simulink model "template_inverted_pendulum_2021b"  (R2021b)
settings: Solver=FixedStepDiscrete  StartTime=0.0  StopTime=inf  FixedStep=0.005  RelTol=1e-3
values from neighbouring files (symbols this model uses):
  LPF_A = [0              1           0               0 ... (first row only)    [IP_experiment.m]    (also in IP_sim.m)
  LPF_B = [                    0                           0 ... (first row only)    [IP_experiment.m]    (also in IP_sim.m)
  LPF_C = [-1/T_s    1/T_s         0         0 ... (first row only)    [IP_experiment.m]    (also in IP_sim.m)
  LPF_D = zeros(2)    [IP_experiment.m]    (also in IP_sim.m)
  rnd = randi(500, 1)    [IP_experiment.m]    (also in IP_sim.m)
  xd = [0.3          0.0      0   0]'    [IP.m]    (also in IP_experiment.m = [0.0    0.0]; IP_sim.m = sp(1:12800, 1))
undefined symbols (not defined in the file or in its folder): K, National_Instruments, PCI
libraries: sldrtlib x2, simulink_extras x1
settings Model: SimulationMode=external  ExtModeTrigDuration=200000  Creator=magudelo  LastModifiedBy=yz
settings SolverCC: AlgebraicLoopSolver=TrustRegion  InsertRTBMode=Always
settings DataIOCC: LimitDataPoints=on  SaveFormat=Array  SignalLoggingSaveFormat=ModelDataLogs  ReturnWorkspaceOutputs=off
settings OptimizationCC: ExpressionDepthLimit=2147483647
settings DebuggingCC: UnderspecifiedInitializationDetection=Classic  MergeDetectMultiDrivingBlocksExec=none  SolverPrmCheckMsg=warning  FcnCallInpInsideContextMsg=warning  StateNameClashWarn=warning  SFUnexpectedBacktrackingDiag=warning  SFNoUnconditionalDefaultTransitionDiag=warning  SFExecutionAtInitializationDiag=none  SFMachineParentedDataDiag=warning  ArithmeticOperatorsInVariantConditions=warning
settings ModelReferenceCC: PropagateSignalLabelsOutOfModel=off
settings SFSimCC: SimUseLocalCustomCode=off  CustomCodeUndefinedFunction=UseInterfaceOnly
settings RTWCC: Description=Simulink Desktop Real-Time  SystemTargetFile=sldrt.tlc  TemplateMakefile=sldrt.tmf  RTWUseLocalCustomCode=off  RTWCompilerOptimization=on
settings CodeAppCC: MaxIdLength=95  StateflowObjectComments=on
settings SimulinkDesktopRealTimeCC: TargetPreCompLibLocation=C:\Program Files\MATLAB\R2021b\toolbox\sldrt\lib\win64  TargetLangStandard=C89/C90 (ANSI)  SupportVariableSizeSignals=off
settings ConfigComp: CovMetricSettings=dw  CovSaveCumulativeToWorkspaceVar=on  CovSaveSingleToWorkspaceVar=on  CovExternalEMLEnable=off

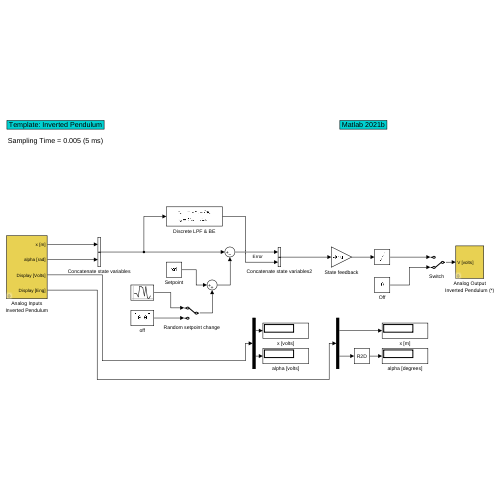
[thumbnail: Simulink's stored preview of the top-level diagram]
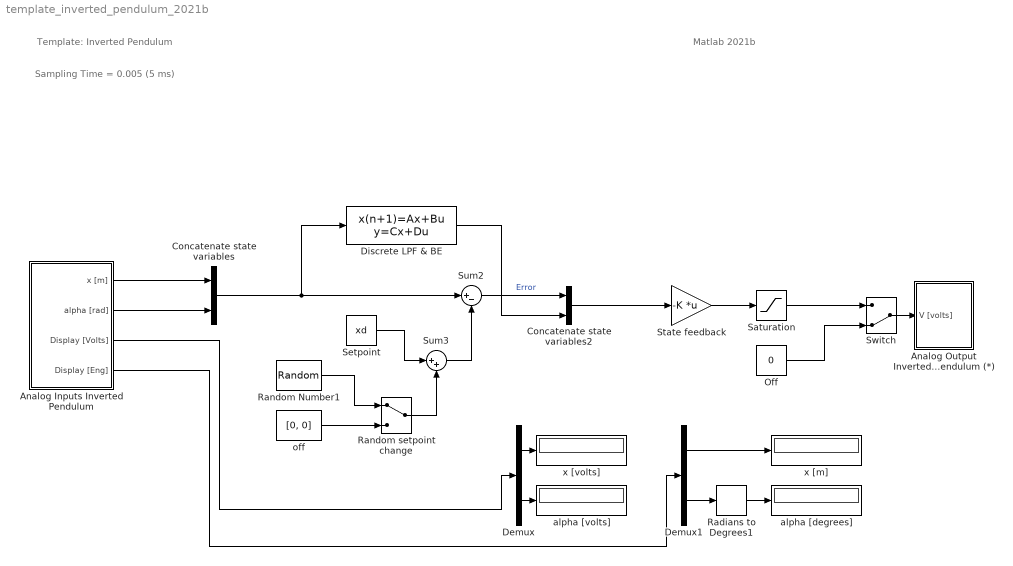
== system template_inverted_pendulum_2021b ==
  note: Matlab 2021b
  note: Template: Inverted Pendulum
  note: Sampling Time = 0.005 (5 ms)
  Analog Inputs Inverted Pendulum : Subsystem  mask(Analog Inputs. Inverted Pendulum){v2m=0.1033, offset_x=0, v2r=0.2482, offset_alfa=0.17011}
      mask prompts: v2m "F_x = Convertion factor from Volts to Meters:"; offset_x "Off_x = Offset for the Cart Position [Volts] :"; v2r "F_alpha = Convertion Factor from Volts to Radians :"; offset_alfa "Off_alpha = Offset for the angle of the rob [Volts] :"
      mask help:
      | Remember:
      |    Cart Position (x)           => channel ACH0
      |    Angle of the rod (alpha) => channel ACH1
      |
      |   Cart Position [m] = F_x * ( Cart Position [v] + off_x )
      |   Angle of the rod [rad] = F_alpha * ( Angle of the rod [v] + off_alpha )
  Analog Output Inverted Pendulum (*) : Subsystem  mask(Analog Output - Inverted Pendulum){}
      mask help:
      | Remember
      |    AO 0 => Power Amplifier + Motor
  Concatenate state variables : Concatenate
  Concatenate state variables2 : Concatenate
  Demux : Demux  Outputs=2
  Demux1 : Demux  Outputs=2
  Discrete LPF & BE : DiscreteStateSpace  A=LPF_A  B=LPF_B  C=LPF_C  D=LPF_D  InitialCondition=[0,0,0,0]  SampleTime=-1
  Off : Constant  Value=0
  Radians to Degrees1 : simulink_extras/Transformations/Radians to Degrees
  Random Number1 : RandomNumber  Mean=[0, 0]  Variance=[0.01, 0]  Seed=rnd  SampleTime=8
  Random setpoint change : ManualSwitch
  Saturation : Saturate  UpperLimit=5  LowerLimit=-5
  Setpoint : Constant  Value=xd
  State feedback : Gain  Gain=-K  Multiplication=Matrix(K*u)
  Sum2 : Sum  Inputs=|+-
  Sum3 : Sum  Inputs=|++
  "Switch  " : ManualSwitch  CurrentSetting=0
  alpha [degrees] : Display
  alpha [volts] : Display
  off : Constant  Value=[0, 0]
  x [m] : Display
  x [volts] : Display
  wires:
  Off/1 -> "Switch  "/2
  Demux/1 -> x [volts]/1
  Demux1/1 -> x [m]/1
  Demux1/2 -> Radians to Degrees1/1
  Radians to Degrees1/1 -> alpha [degrees]/1
  Analog Inputs Inverted Pendulum/4(Display [Eng]) -> Demux1/1
  Demux/2 -> alpha [volts]/1
  Analog Inputs Inverted Pendulum/3(Display [Volts]) -> Demux/1
  Analog Inputs Inverted Pendulum/1(x [m]) -> Concatenate state variables/1
  Concatenate state variables/1 -> Discrete LPF & BE/1, Sum2/1
  Random setpoint change/1 -> Sum3/2
  off/1 -> Random setpoint change/2
  Setpoint/1 -> Sum3/1
  Random Number1/1 -> Random setpoint change/1
  Sum2/1 -> Concatenate state variables2/1  "Error"
  Sum3/1 -> Sum2/2
  Discrete LPF & BE/1 -> Concatenate state variables2/2
  Concatenate state variables2/1 -> State feedback/1
  "Switch  "/1 -> Analog Output Inverted Pendulum (*)/1(V [volts])
  Analog Inputs Inverted Pendulum/2(alpha [rad]) -> Concatenate state variables/2
  Saturation/1 -> "Switch  "/1
  State feedback/1 -> Saturation/1

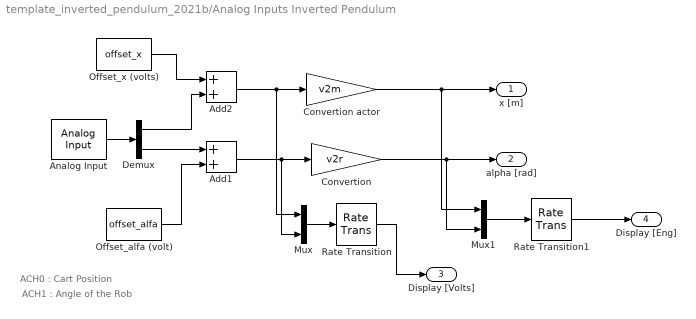
== system template_inverted_pendulum_2021b/Analog Inputs Inverted Pendulum ==
  note: ACH0 : Cart Position
  note: ACH1 : Angle of the Rob
  Add1 : Sum
  Add2 : Sum
  Analog Input : sldrtlib/Analog Input  SampleTime=0.005  MaxMissedTicks=10  ShowMissedTicks=off  YieldWhenWaiting=off  DrvName=National_Instruments/PCI-6014  DrvAddress=4294967295  DrvOptions=[1 0 0 0 0 0]  Channels=[1 2]  RangeMode=1  VoltRange=1  DataType=1
      settings: AttributesFormatString=National Instruments\nPCI-6014 [auto]
  "Convertion " : Gain  Gain=v2r
  Convertion actor : Gain  Gain=v2m
  Demux : Demux  Outputs=2
  Mux : Mux  Inputs=2
  Mux1 : Mux  Inputs=2
  Offset_alfa (volt) : Constant  Value=offset_alfa
  Offset_x (volts) : Constant  Value=offset_x
  Rate Transition : RateTransition  OutPortSampleTime=0.25
  Rate Transition1 : RateTransition  OutPortSampleTime=0.25
  x [m] : Outport  VectorParamsAs1DForOutWhenUnconnected=off
  alpha [rad] : Outport  Port=2  VectorParamsAs1DForOutWhenUnconnected=off
  Display [Volts] : Outport  Port=3  VectorParamsAs1DForOutWhenUnconnected=off
  Display [Eng] : Outport  Port=4  VectorParamsAs1DForOutWhenUnconnected=off
  wires:
  Analog Input/1 -> Demux/1
  Demux/1 -> Add2/2
  Add2/1 -> Convertion actor/1, Mux/1
  Offset_x (volts)/1 -> Add2/1
  Convertion actor/1 -> x [m]/1, Mux1/1
  Demux/2 -> Add1/1
  Offset_alfa (volt)/1 -> Add1/2
  Add1/1 -> "Convertion "/1, Mux/2
  "Convertion "/1 -> alpha [rad]/1, Mux1/2
  Mux/1 -> Rate Transition/1
  Rate Transition/1 -> Display [Volts]/1
  Mux1/1 -> Rate Transition1/1
  Rate Transition1/1 -> Display [Eng]/1

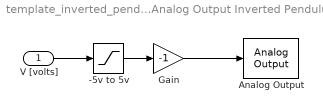
== system template_inverted_pendulum_2021b/Analog Output Inverted Pendulum (*) ==
  V [volts] : Inport
  -5v to 5v : Saturate  UpperLimit=5  LowerLimit=-5
  Analog Output : sldrtlib/Analog Output  SampleTime=0.005  MaxMissedTicks=10  ShowMissedTicks=off  YieldWhenWaiting=off  DrvName=National_Instruments/PCI-6014  DrvAddress=4294967295  DrvOptions=[1 0 0 0 0 0]  Channels=1  RangeMode=1  VoltRange=1  InitialValue=0  FinalValue=0
      settings: AttributesFormatString=National Instruments\nPCI-6014 [auto]
  Gain : Gain  Gain=-1
  wires:
  -5v to 5v/1 -> Gain/1
  V [volts]/1 -> -5v to 5v/1
  Gain/1 -> Analog Output/1
